simulink model "FSM"  (R2023b)
settings: configuration reference "Configuration" (kept outside this file)
settings Model: Creator=leona  LastModifiedBy=leona
settings ConfigSetRef: SourceName=Configuration  SourceLocation=Base Workspace

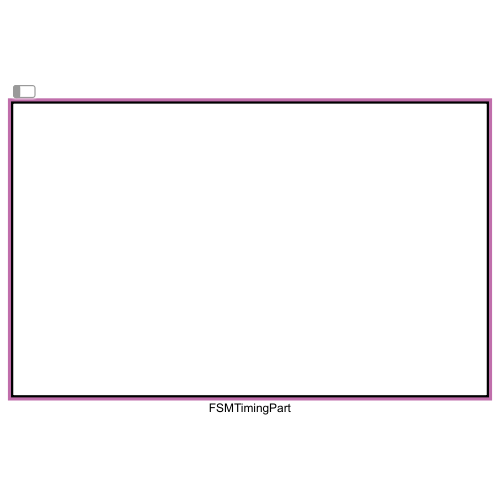
[thumbnail: Simulink's stored preview of the top-level diagram]
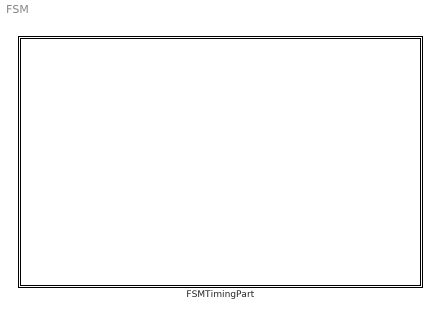
== system FSM ==
  FSMTimingPart : Subsystem  TreatAsAtomicUnit=on  ScheduleAs=Periodic partition  PartitionName=FSMTimingPart  SystemSampleTime=0.05

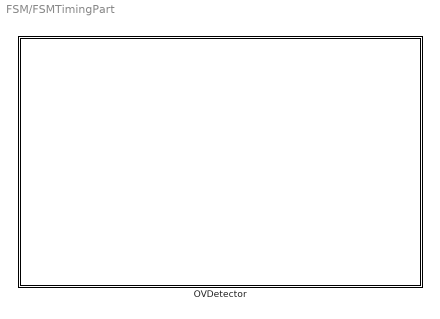
== system FSM/FSMTimingPart ==
  OVDetector : Stateflow chart  TreatAsAtomicUnit=on

== stateflow chart FSM/FSMTimingPart/OVDetector ==
  state STATE_TSON
    SMKACADEMY.fsm.state = TS_ON;
    SMKACADEMY.electrical.switch_state = SWITCH_CLOSED;
  state STATE_PRECHARGE
    SMKACADEMY.fsm.state = PRECHARGE;
    SMKACADEMY.electrical.switch_state = SWITCH_PRECHARGE;
    SMKACADEMY.fsm.tPrecharge++;
  state STATE_TSOFF
    SMKACADEMY.fsm.state = TS_OFF;
    SMKACADEMY.electrical.switch_state = SWITCH_DISCHARGE;
  state STATE_FAULT
    SMKACADEMY.fsm.state = FAULT;
  (junction 21) -> (junction 20)
  (junction 22) -> (junction 21)
  (junction 20) -> STATE_TSOFF
  STATE_PRECHARGE -> (junction 21) [order 3] : [hasChangedTo(SMKACADEMY.fsm.hw_switch, 1) || SMKACADEMY.fsm.tPrecharge > 140]
  STATE_TSON -> (junction 22) [order 2] : [hasChangedTo(SMKACADEMY.fsm.hw_switch, 1)]
  (default) -> STATE_TSOFF
  STATE_TSOFF -> STATE_PRECHARGE [order 2] : [hasChangedTo(SMKACADEMY.fsm.hw_switch, 1)]
      | {SMKACADEMY.fsm.tPrecharge = 0;}
  STATE_PRECHARGE -> STATE_TSON [order 2] : [SMKACADEMY.fsm.tPrecharge > 100 && (SMKACADEMY.electrical.vTSAcc > (0.95f * SMKACADEMY.electrical.vSumOfCells))]
  STATE_TSOFF -> (junction 11) [order 1] : [SMKACADEMY.electrical.vTSAcc > 600]
  STATE_PRECHARGE -> (junction 14) [order 1] : [SMKACADEMY.electrical.vTSAcc > 600]
  STATE_TSON -> (junction 15) [order 1] : [SMKACADEMY.electrical.vTSAcc > 600]
  (junction 14) -> (junction 11)
  (junction 15) -> (junction 14)
  (junction 11) -> STATE_FAULT
  data: SMKACADEMY data_store_memory
